simulink model "Simulation_der_Regler"  (R2016a)
settings: Solver=FixedStepAuto  StartTime=0  StopTime=10.0  FixedStep=T_s  RelTol=1e-3
values from neighbouring files (symbols this model uses):
  AD1 = expm(AC1*T_s)    [Regerlung_einer_WEA.m]
  AD2 = expm(AC2*T_s)    [Regerlung_einer_WEA.m]
  AD4 = expm(AC4*T_s)    [Regerlung_einer_WEA.m]
  BD1 = inv(AC1)*(expm(AC1*T_s)-I1)*BC1    [Regerlung_einer_WEA.m]
  BD2 = inv(AC2)*(expm(AC2*T_s)-I2)*BC2    [Regerlung_einer_WEA.m]
  BD2u = BD2(:,1:2)    [Regerlung_einer_WEA.m]
  BD4 = inv(AC4)*(expm(AC4*T_s)-I4)*BC4    [Regerlung_einer_WEA.m]
  C1 = zeors(s1*Nu,s1)    [OptimierungMitConstrains.m]    (also in Regerlung_einer_WEA.m = 1)
  C2 = zeors(s1*Nu,s1*Nu)    [OptimierungMitConstrains.m]    (also in Regerlung_einer_WEA.m = [1,0,0,0])
  C2full = eye(4)    [Regerlung_einer_WEA.m]
  C4 = [1,0,0,0,0,0,0,0 ... (first row only)    [Regerlung_einer_WEA.m]
  C4_base = [1,0,0,0,0,0,0,0 ... (first row only)    [Regerlung_einer_WEA.m]
  D1 = zeros(1,3)    [Regerlung_einer_WEA.m]
  D2 = zeros(1,3)    [Regerlung_einer_WEA.m]
  D2full = zeros(4,3)    [Regerlung_einer_WEA.m]
  D4 = zeros(5,3)    [Regerlung_einer_WEA.m]
  D4_base = zeros(6,3)    [Regerlung_einer_WEA.m]
  DeltaU2max = [8+pi/180+T_s,Inf]    [Regerlung_einer_WEA.m]
  DeltaU2min = [-8*pi/180*T_s,-Inf]    [Regerlung_einer_WEA.m]
  para_cntrl = struct()    [create_para_cntrl_5MWBaseline.m]    (also in para_cntrl_5MWBaseline.mat = )
  para_mdl = struct()    [Regerlung_einer_WEA.m]
  Qw2 = eye(100)*0.1    [Regerlung_einer_WEA.m]
  r2 = zeros(1,100)    [Regerlung_einer_WEA.m]
  ref_4 = [w_r_c;0;y_t_c;0;y_b_c]    [Regerlung_einer_WEA.m]
  Rw2 = eye(100)    [Regerlung_einer_WEA.m]
  T_g_c = 43093.5    [Regerlung_einer_WEA.m]
  T_s = 0.05    [Regerlung_einer_WEA.m]
  theta_c = 4*pi/180    (= 0.0698131700798)    [Regerlung_einer_WEA.m]
  U2max = [90*pi/180,43091.5]    [Regerlung_einer_WEA.m]
  U2min = [0,0]    [Regerlung_einer_WEA.m]
  v_c = 14.0    (= 14)    [Regerlung_einer_WEA.m]    (also in testinterpolation.m = [9,9.5,10,11,14,15,18,25])
  w_g_c = w_r_c*n_g    (= 122.9087)    [Regerlung_einer_WEA.m]
  w_r_c = 1.2671    [Regerlung_einer_WEA.m]
  Y2max = Inf    (= inf)    [Regerlung_einer_WEA.m]
  Y2min = 0    [Regerlung_einer_WEA.m]
  y_b_c = Datalogging.yb(s1(1))    [Regerlung_einer_WEA.m]
  y_t_c = Datalogging.yt(s1(1))    [Regerlung_einer_WEA.m]
undefined symbols (not defined in the file or in its folder): BD2ua, F2, F2a, G2, G2a, H2, H2a, v_t_c
libraries: mpclib x6
settings Model: Creator=pasca  LastModifiedBy=pasca
settings GRTTargetCC: GeneratePreprocessorConditionals=Use local settings

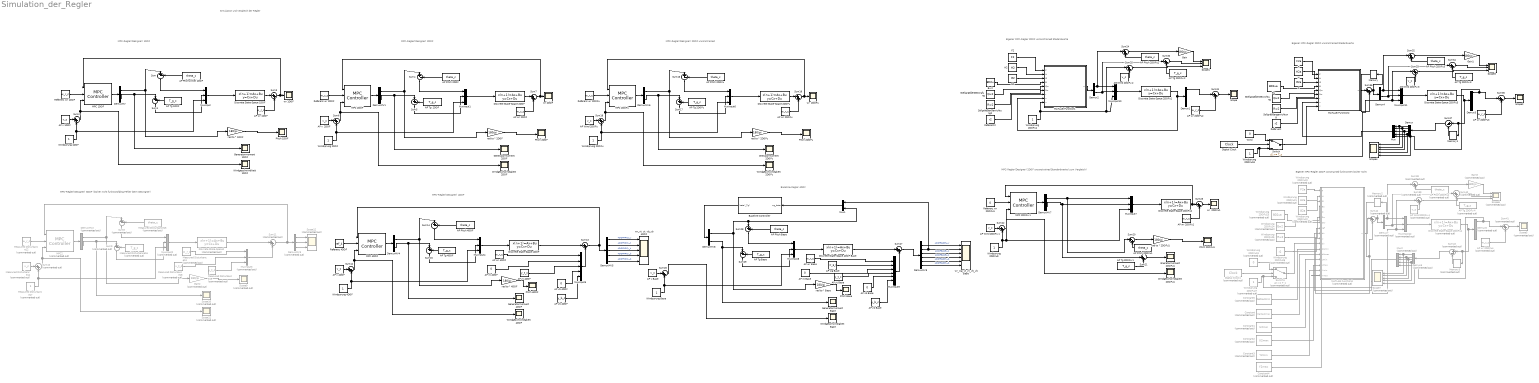
== system Simulation_der_Regler ==
  note: Eigener MPC-Regler 2DOF unconstrained Stadardwerte
  note: Simulation und Vergleich der Regler
  note: Baseline-Regler 4DOF
  note: MPC-Regler(Designer) 1DOF
  note: MPC-Regler(Designer) 2DOF
  note: MPC-Regler(Designer) 3DOF (bisher nicht funktionsfähig Fehler beim Desingner)
  note: MPC-Regler(Designer) 4DOF
  note: MPC-Regler(Designer) 2DOF unconstrained
  note: MPC-Regler(Designer) 2DOF unconstrained Standardwerte (zum Vergleich)
  note: Eigener MPC-Regler 2DOF unconstrained Stadardwerte
  note: Eigener MPC-Regler 2DOF constrained funktioniert bisher nicht
  " AP Ptichwinkel 1DOF " : Constant  Value=theta_c
  "AP Pitch 2DOF " : Constant  Value=theta_c
  AP Pitch 2DOFu{,1..3} (4 alike) : Constant  Value=theta_c
  AP Pitch 2DOFu4 : Constant  Commented=on  Value=theta_c
  AP Pitch 4DOF : Constant  Value=theta_c
  AP Pitch Base : Constant  Value=theta_c
  AP Tg  2DOF : Constant  Value=T_g_c
  "AP Tg 1DOF " : Constant  Value=T_g_c
  AP Tg 2DOFu {,1..3} (4 alike) : Constant  Value=T_g_c
  AP Tg 2DOFu 4 : Constant  Commented=on  Value=T_g_c
  AP Tg 4DOF : Constant  Value=T_g_c
  AP Tg Base : Constant  Value=T_g_c
  AP Wind 2DOFu {,1..3} (4 alike) : Constant  Value=v_c
  AP Wind 2DOFu 4 : Constant  Commented=on  Value=v_c
  AP v  2DOF : Constant  Value=v_c
  AP v 1DOF : Constant  Value=v_c
  "AP v 4DOF " : Constant  Value=v_c
  AP v Base : Constant  Value=v_c
  AP vb 4DOF : Constant  Value=0
  AP vb Base : Constant  Value=0
  AP vt 4DOF : Constant  Value=0
  AP vt Base : Constant  Value=0
  AP wg Base : Constant  Value=w_g_c
  "AP wr 1DOF " : Constant  Value=w_r_c
  "AP wr 2DOF " : Constant  Value=w_r_c
  AP wr 2DOFu{,1..3} (4 alike) : Constant  Value=w_r_c
  AP wr 2DOFu4 : Constant  Commented=on  Value=w_r_c
  AP wr 4DOF : Constant  Value=w_r_c
  AP wr Base : Constant  Value=w_r_c
  AP yb 4DOF : Constant  Value=y_b_c
  AP yb Base : Constant  Value=y_b_c
  AP yt 4DOF : Constant  Value=y_t_c
  AP yt Base : Constant  Value=y_t_c
  Baseline Controller : Subsystem
  "Bu " : Constant  Value=BD2ua
  Bu 2 : Constant  Value=BD2u
  Constant : Constant  Commented=on  Value=DeltaU2max
  Constant1 : Constant  Commented=on  Value=U2min
  Constant2 : Constant  Commented=on  Value=U2max
  Constant3 : Constant  Commented=on  Value=Y2min
  Constant4 : Constant  Commented=on  Value=Y2max
  Constant5 : Constant  Commented=on  Value=DeltaU2min
  Demux : Demux
  Demux1 : Demux
  Demux2 : Demux  Outputs=2
  Demux3 : Demux
  Demux4 : Demux  Outputs=2
  Demux5 : Demux  Commented=on
  Demux6 : Demux  Commented=on
  Demux7 : Demux  Commented=on  Outputs=2
  DemuxMV{,1,4,6..8} (6 alike) : Demux  Outputs=2
  DemuxMV2 : Demux  Commented=on  Outputs=2
  DemuxMV3 : Demux  Commented=on  Outputs=3
  DemuxMV5 : Demux  Outputs=5
  DemuxMV9 : Demux  Outputs=6
  Digital Clock : DigitalClock  SampleTime=T_s
  Digital Clock1 : DigitalClock  Commented=on  SampleTime=T_s
  "Discrete State-Space 1DOF " : DiscreteStateSpace  A=AD1  B=BD1  C=C1  D=D1  SampleTime=T_s
  Discrete State-Space 2DOF : DiscreteStateSpace  A=AD2  B=BD2  C=C2  D=D2  SampleTime=T_s
  Discrete State-Space 2DOFu : DiscreteStateSpace  A=AD2  B=BD2  C=C2  D=D2  SampleTime=T_s
  Discrete State-Space 2DOFu1 : DiscreteStateSpace  A=AD2  B=BD2  C=C2full  D=D2full  SampleTime=T_s
  Discrete State-Space 2DOFu2 : DiscreteStateSpace  A=AD2  B=BD2  C=C2  D=D2  SampleTime=T_s
  Discrete State-Space 2DOFu3 : DiscreteStateSpace  A=AD2  B=BD2  C=C2full  D=D2full  SampleTime=T_s
  Discrete State-Space 2DOFu4 : DiscreteStateSpace  Commented=on  A=AD2  B=BD2  C=C2full  D=D2full  SampleTime=T_s
  Discrete State-Space 4DOF : DiscreteStateSpace  A=AD4  B=BD4  C=C4  D=D4  SampleTime=T_s
  Discrete State-Space 4DOF Base : DiscreteStateSpace  A=AD4  B=BD4  C=C4_base  D=D4_base  SampleTime=T_s
  Discrete State-Space2 : DiscreteStateSpace  Commented=on  A=AD2  B=BD2  C=C2  D=D2  SampleTime=T_s
  "F " : Constant  Value=F2a
  F2 : Constant  Value=F2
  "G " : Constant  Value=G2a
  "G2 " : Constant  Value=G2
  Gain : Gain  Gain=180/pi
  Gain1 : Gain  Gain=180/pi
  Gain2 : Gain  Commented=on  Gain=180/pi
  Gain3 : Gain  Commented=on  Gain=180/pi
  "Generatormoment 1DOF " : Scope
  "Generatormoment 2DOF " : Scope
  Generatormoment 4DOF : Scope
  Generatormoment Base : Scope
  Gneratormoment 2DOFu : Scope
  Gneratormoment 2DOFu1 : Scope
  "H " : Constant  Value=H2a
  "H2 " : Constant  Value=H2
  MATLAB Function1 : MATLAB Function  TreatAsAtomicUnit=on
  MATLAB Function2 : MATLAB Function  TreatAsAtomicUnit=on
  MATLAB Function3 : MATLAB Function  Commented=on  TreatAsAtomicUnit=on
  "MPC 1DOF " : mpclib/MPC Controller  SCDEnableBlockLinearizationSpecification=on  mpcobj=mpc_F1  is_multiple=0  enable_value=0  return_u0=off  ref_from_ws=off  ref_signal_name=[]  ref_preview=off  md_from_ws=off  md_signal_name=[]  md_preview=off  from_project=off  project_file=MPCtask.mat  md_inport=on  mv_inport=off  cost_outport=off  return_sequence=off  return_qpstatus=off  return_state=off  state_inport=off  lims_inport=off  ywt_inport=off  is_designfromscratch=0  uwt_inport=off  duwt_inport=off  rhoeps_inport=off  uref_inport=off  n_ts=0.05  n_mv=2  n_md=1  n_ud=0  n_mo=1  n_uo=0  BlockDataType=double  SampleTimeInherited=off  switch_inport=off
  "MPC 2DOF " : mpclib/MPC Controller  SCDEnableBlockLinearizationSpecification=on  mpcobj=mpc_F2  is_multiple=0  enable_value=0  return_u0=off  ref_from_ws=off  ref_signal_name=[]  ref_preview=off  md_from_ws=off  md_signal_name=[]  md_preview=off  from_project=off  project_file=MPCtask.mat  md_inport=on  mv_inport=off  cost_outport=off  return_sequence=off  return_qpstatus=off  return_state=off  state_inport=off  lims_inport=off  ywt_inport=off  is_designfromscratch=0  uwt_inport=off  duwt_inport=off  rhoeps_inport=off  uref_inport=off  n_ts=0.05  n_mv=2  n_md=1  n_ud=0  n_mo=1  n_uo=0  BlockDataType=double  SampleTimeInherited=off  switch_inport=off
  "MPC 2DOFu " : mpclib/MPC Controller  SCDEnableBlockLinearizationSpecification=on  mpcobj=mpc_F2_u  is_multiple=0  enable_value=0  return_u0=off  ref_from_ws=off  ref_signal_name=[]  ref_preview=off  md_from_ws=off  md_signal_name=[]  md_preview=off  from_project=off  project_file=MPCtask.mat  md_inport=on  mv_inport=off  cost_outport=off  return_sequence=off  return_qpstatus=off  return_state=off  state_inport=off  lims_inport=off  ywt_inport=off  is_designfromscratch=0  uwt_inport=off  duwt_inport=off  rhoeps_inport=off  uref_inport=off  n_ts=0.05  n_mv=2  n_md=1  n_ud=0  n_mo=1  n_uo=0  BlockDataType=double  SampleTimeInherited=off  switch_inport=off
  MPC 2DOFu 1 : mpclib/MPC Controller  SCDEnableBlockLinearizationSpecification=on  mpcobj=mpc_F2_us  is_multiple=0  enable_value=0  return_u0=off  ref_from_ws=off  ref_signal_name=[]  ref_preview=off  md_from_ws=off  md_signal_name=[]  md_preview=off  from_project=off  project_file=MPCtask.mat  md_inport=on  mv_inport=off  cost_outport=off  return_sequence=off  return_qpstatus=off  return_state=off  state_inport=off  lims_inport=off  ywt_inport=off  is_designfromscratch=0  uwt_inport=off  duwt_inport=off  rhoeps_inport=off  uref_inport=off  n_ts=0.05  n_mv=2  n_md=1  n_ud=0  n_mo=1  n_uo=0  BlockDataType=double  SampleTimeInherited=off  switch_inport=off
  MPC 4DOF : mpclib/MPC Controller  SCDEnableBlockLinearizationSpecification=on  mpcobj=mpc_F4  is_multiple=0  enable_value=0  return_u0=off  ref_from_ws=off  ref_signal_name=[]  ref_preview=off  md_from_ws=off  md_signal_name=[]  md_preview=off  from_project=off  project_file=MPCtask.mat  md_inport=on  mv_inport=off  cost_outport=off  return_sequence=off  return_qpstatus=off  return_state=off  state_inport=off  lims_inport=off  ywt_inport=off  is_designfromscratch=0  uwt_inport=off  duwt_inport=off  rhoeps_inport=off  uref_inport=off  n_ts=0.05  n_mv=2  n_md=1  n_ud=0  n_mo=5  n_uo=0  BlockDataType=double  SampleTimeInherited=off  switch_inport=off
  MPC2 : mpclib/MPC Controller  Commented=on  SCDEnableBlockLinearizationSpecification=on  mpcobj=mpc_F1  is_multiple=0  enable_value=0  return_u0=off  ref_from_ws=off  ref_signal_name=[]  ref_preview=off  md_from_ws=off  md_signal_name=[]  md_preview=off  from_project=off  project_file=MPCtask.mat  md_inport=on  mv_inport=off  cost_outport=off  return_sequence=off  return_qpstatus=off  return_state=off  state_inport=off  lims_inport=off  ywt_inport=off  is_designfromscratch=0  uwt_inport=off  duwt_inport=off  rhoeps_inport=off  uref_inport=off  n_ts=0.05  n_mv=2  n_md=1  n_ud=0  n_mo=1  n_uo=0  BlockDataType=double  SampleTimeInherited=off  switch_inport=off
  Measured Disturbance12 : Constant  Commented=on  Value=w_r_c
  Measured Disturbance13 : Constant  Commented=on  Value=w_r_c
  Measured Disturbance14 : Constant  Commented=on  Value=v_c
  Measured Disturbance15 : Constant  Commented=on  Value=theta_c
  Measured Disturbance16 : Constant  Commented=on  Value=T_g_c
  Measured Disturbance17 : Constant  Commented=on
  Measured Disturbance18 : Constant  Commented=on  Value=v_t_c
  Measured Disturbance19 : Constant  Commented=on  Value=y_t_c
  Memory : Memory
  Memory1 : Memory
  Memory2 : Memory  Commented=on
  Memory3 : Memory  Commented=on
  Mux : Mux  Inputs=5
  Mux1 : Mux  Inputs=2
  Mux2 : Mux  Commented=on  Inputs=5
  MuxInput{,1,4,6..8,10..11} (8 alike) : Mux  Inputs=3
  MuxInput12 : Mux  Commented=on  Inputs=3
  MuxInput2 : Mux  Commented=on  Inputs=3
  MuxInput3 : Mux  Commented=on  Inputs=3
  MuxInput5 : Mux  Inputs=5
  MuxInput9 : Mux  Inputs=6
  "Pitch 1DOF " : Scope
  Pitch 2DOFu : Scope
  Pitch 2DOFu1 : Scope
  Pitch 4DOF : Scope
  Pitch Base : Scope
  "Ptich 2DOF " : Scope
  Refer enz : Constant  Value=r2
  Referenz 4DOF : Constant  Value=ref_4
  "Referenz wr 1DOF " : Constant  Value=w_r_c
  "Referenz wr 2DOF " : Constant  Value=w_r_c
  Referenz wr 2DOFu : Constant  Value=w_r_c
  Referenz wr 2DOFu1 : Constant  Value=0
  "Referenz2 " : Constant  Value=r2
  Scope : Scope
  Scope1 : Scope  NumInputPorts=3
  Scope{5,9..11} (4 alike) : Scope  Commented=on
  Scope12 : Scope  Commented=on  NumInputPorts=3
  Scope2 : Scope
  Scope3 : Scope  NumInputPorts=3
  Scope4 : Scope  NumInputPorts=5
  Scope6 : Scope  Commented=on  NumInputPorts=3
  Scope7 : Scope  Commented=on  NumInputPorts=5
  SollgräößenGewichtung2 : Constant  Value=Rw2
  Sollgräößengewichtung : Constant  Value=Rw2
  StellgräößenBestrafung : Constant  Value=Qw2
  "StellgräößenGewichtung " : Constant  Value=Qw2
  Sum{,1,4..5,14..17,28..29,37} (11 alike) : Sum  Inputs=|+-
  Sum{10..11,38..42} (7 alike) : Sum  Commented=on  Inputs=|++
  Sum{2..3,6..7,12..13,18..27,30..36} (23 alike) : Sum  Inputs=|++
  Sum43 : Sum  Commented=on  Inputs=|+-
  Sum8 : Sum  Commented=on  Inputs=|+-
  Sum9 : Sum  Commented=on  Inputs=|+-
  Switch : Switch  Threshold=T_s
  Switch1 : Switch  Commented=on  Threshold=T_s
  "Wind " : Constant  Value=0  VectorParams1D=off  SampleTime=T_s
  "Windgeschwindigkeit 2DOF " : Scope
  Windgeschwindigkeit 2DOFu : Scope
  Windgeschwindigkeit 2DOFu1 : Scope
  Windgeschwindigkeit 4DOF : Scope
  Windgeschwindigkeit Base : Scope
  "Windgeschwindikeit 1DOF " : Scope
  "Windsprung 1DOF " : Constant
  "Windsprung 2DOF " : Constant
  Windsprung 2DOFu : Constant
  Windsprung 2DOFu1 : Constant
  Windsprung 2DOFu18 : Constant  VectorParams1D=off  SampleTime=T_s
  Windsprung 2DOFu19 : Constant  Commented=on  Value=0  VectorParams1D=off  SampleTime=T_s
  Windsprung 2DOFu20 : Constant  Commented=on  Value=F2a
  Windsprung 2DOFu21 : Constant  Commented=on  Value=H2a
  Windsprung 2DOFu22 : Constant  Commented=on  Value=G2a
  Windsprung 2DOFu23 : Constant  Commented=on  Value=BD2ua
  Windsprung 2DOFu24 : Constant  Commented=on  Value=Qw2
  Windsprung 2DOFu25 : Constant  Commented=on  Value=Rw2
  Windsprung 2DOFu26 : Constant  Commented=on  Value=r2
  Windsprung 2DOFu27 : Constant  Commented=on  VectorParams1D=off  SampleTime=T_s
  Windsprung 2DOFu9 : Constant
  Windsprung 4DOF : Constant
  Windsprung Base : Constant
  "rad to ° 1DOF " : Gain  Gain=180/pi
  "rad to ° 2DOF " : Gain  Gain=180/pi
  rad to ° 2DOFu : Gain  Gain=180/pi
  rad to ° 2DOFu1 : Gain  Gain=180/pi
  rad to ° 4DOF : Gain  Gain=180/pi
  rad to ° Base : Gain  Gain=180/pi
  wr  2DOFu : Scope
  wr  2DOFu1 : Scope
  "wr 1DOF " : Scope
  wr 2DOF : Scope
  wr_vt_yt_vb_yb 4DOF : Scope  NumInputPorts=5
  wr_wg_vt_yt_vb_yb Base : Scope  NumInputPorts=6
  wires:
  "Referenz wr 1DOF "/1 -> "MPC 1DOF "/2
  "MPC 1DOF "/1 -> DemuxMV/1
  MuxInput/1 -> "Discrete State-Space 1DOF "/1
  Sum/1 -> MuxInput/1
  DemuxMV/1 -> Sum/1, "rad to ° 1DOF "/1
  " AP Ptichwinkel 1DOF "/1 -> Sum/2
  DemuxMV/2 -> "Generatormoment 1DOF "/1, Sum1/1
  Sum1/1 -> MuxInput/2
  "AP Tg 1DOF "/1 -> Sum1/2
  AP v 1DOF/1 -> Sum2/1
  Sum2/1 -> "Windgeschwindikeit 1DOF "/1, "MPC 1DOF "/3
  "Windsprung 1DOF "/1 -> MuxInput/3, Sum2/2
  "Discrete State-Space 1DOF "/1 -> Sum3/1
  "AP wr 1DOF "/1 -> Sum3/2
  Sum3/1 -> "wr 1DOF "/1, "MPC 1DOF "/1
  "rad to ° 1DOF "/1 -> "Pitch 1DOF "/1
  "Referenz wr 2DOF "/1 -> "MPC 2DOF "/2
  "MPC 2DOF "/1 -> DemuxMV1/1
  MuxInput1/1 -> Discrete State-Space 2DOF/1
  Sum4/1 -> MuxInput1/1
  DemuxMV1/1 -> Sum4/1, "rad to ° 2DOF "/1
  "AP Pitch 2DOF "/1 -> Sum4/2
  DemuxMV1/2 -> "Generatormoment 2DOF "/1, Sum5/1
  Sum5/1 -> MuxInput1/2
  AP Tg  2DOF/1 -> Sum5/2
  AP v  2DOF/1 -> Sum6/1
  Sum6/1 -> "Windgeschwindigkeit 2DOF "/1, "MPC 2DOF "/3
  "Windsprung 2DOF "/1 -> MuxInput1/3, Sum6/2
  Discrete State-Space 2DOF/1 -> Sum7/1
  "AP wr 2DOF "/1 -> Sum7/2
  Sum7/1 -> wr 2DOF/1, "MPC 2DOF "/1
  "rad to ° 2DOF "/1 -> "Ptich 2DOF "/1
  Measured Disturbance12/1 -> MPC2/2
  MPC2/1 -> DemuxMV2/1
  MuxInput2/1 -> Discrete State-Space2/1
  Sum8/1 -> MuxInput2/1
  DemuxMV2/1 -> Sum8/1, Gain2/1
  Measured Disturbance15/1 -> Sum8/2
  DemuxMV2/2 -> Scope10/1, Sum9/1
  Sum9/1 -> MuxInput2/2
  Measured Disturbance16/1 -> Sum9/2
  Measured Disturbance14/1 -> Sum10/1
  Sum10/1 -> Scope11/1, MPC2/3
  Measured Disturbance17/1 -> MuxInput2/3, Sum10/2
  Sum11/1 -> DemuxMV3/1, MPC2/1
  Gain2/1 -> Scope9/1
  Discrete State-Space2/1 -> Sum11/1
  MuxInput3/1 -> Sum11/2
  DemuxMV3/1 -> Scope12/1
  DemuxMV3/2 -> Scope12/2
  DemuxMV3/3 -> Scope12/3
  Measured Disturbance13/1 -> MuxInput3/1
  Measured Disturbance19/1 -> MuxInput3/3
  Measured Disturbance18/1 -> MuxInput3/2
  Referenz 4DOF/1 -> MPC 4DOF/2
  MPC 4DOF/1 -> DemuxMV4/1
  MuxInput4/1 -> Discrete State-Space 4DOF/1
  Sum14/1 -> MuxInput4/1
  DemuxMV4/1 -> Sum14/1, rad to ° 4DOF/1
  AP Pitch 4DOF/1 -> Sum14/2
  DemuxMV4/2 -> Generatormoment 4DOF/1, Sum15/1
  Sum15/1 -> MuxInput4/2
  AP Tg 4DOF/1 -> Sum15/2
  "AP v 4DOF "/1 -> Sum12/1
  Sum12/1 -> Windgeschwindigkeit 4DOF/1, MPC 4DOF/3
  Windsprung 4DOF/1 -> MuxInput4/3, Sum12/2
  Sum13/1 -> DemuxMV5/1, MPC 4DOF/1
  rad to ° 4DOF/1 -> Pitch 4DOF/1
  Discrete State-Space 4DOF/1 -> Sum13/1
  MuxInput5/1 -> Sum13/2
  DemuxMV5/2 -> wr_vt_yt_vb_yb 4DOF/2  "4DOFMPCv_t"
  DemuxMV5/3 -> wr_vt_yt_vb_yb 4DOF/3  "4DOFMPCy_t"
  AP wr 4DOF/1 -> MuxInput5/1
  AP yt 4DOF/1 -> MuxInput5/3
  AP vt 4DOF/1 -> MuxInput5/2
  DemuxMV5/4 -> wr_vt_yt_vb_yb 4DOF/4  "4DOFMPCv_b"
  DemuxMV5/5 -> wr_vt_yt_vb_yb 4DOF/5  "4DOFMPCy_b"
  AP vb 4DOF/1 -> MuxInput5/4
  AP yb 4DOF/1 -> MuxInput5/5
  Referenz wr 2DOFu/1 -> "MPC 2DOFu "/2
  "MPC 2DOFu "/1 -> DemuxMV6/1
  MuxInput6/1 -> Discrete State-Space 2DOFu/1
  Sum16/1 -> MuxInput6/1
  DemuxMV6/1 -> Sum16/1, rad to ° 2DOFu/1
  AP Pitch 2DOFu/1 -> Sum16/2
  DemuxMV6/2 -> Gneratormoment 2DOFu/1, Sum17/1
  Sum17/1 -> MuxInput6/2
  "AP Tg 2DOFu "/1 -> Sum17/2
  "AP Wind 2DOFu "/1 -> Sum18/1
  Sum18/1 -> Windgeschwindigkeit 2DOFu/1, "MPC 2DOFu "/3
  Windsprung 2DOFu/1 -> MuxInput6/3, Sum18/2
  Discrete State-Space 2DOFu/1 -> Sum19/1
  AP wr 2DOFu/1 -> Sum19/2
  Sum19/1 -> wr  2DOFu/1, "MPC 2DOFu "/1
  rad to ° 2DOFu/1 -> Pitch 2DOFu/1
  MuxInput8/1 -> Discrete State-Space 4DOF Base/1
  Sum28/1 -> MuxInput8/1
  DemuxMV8/1 -> rad to ° Base/1, Sum28/1, Mux1/2
  AP Pitch Base/1 -> Sum28/2
  DemuxMV8/2 -> Generatormoment Base/1, Sum29/1
  Sum29/1 -> MuxInput8/2
  AP Tg Base/1 -> Sum29/2
  AP v Base/1 -> Sum26/1
  Sum26/1 -> Windgeschwindigkeit Base/1
  Windsprung Base/1 -> MuxInput8/3, Sum26/2
  Sum27/1 -> DemuxMV9/1
  rad to ° Base/1 -> Pitch Base/1
  Discrete State-Space 4DOF Base/1 -> Sum27/1
  MuxInput9/1 -> Sum27/2
  DemuxMV9/1 -> wr_wg_vt_yt_vb_yb Base/1  "4DOFBASEw_r"
  DemuxMV9/2 -> Mux1/1, wr_wg_vt_yt_vb_yb Base/2
  DemuxMV9/3 -> wr_wg_vt_yt_vb_yb Base/3  "4DOFBASEv_t"
  AP wr Base/1 -> MuxInput9/1
  DemuxMV9/4 -> wr_wg_vt_yt_vb_yb Base/4  "4DOFBASEy_t"
  DemuxMV9/5 -> wr_wg_vt_yt_vb_yb Base/5  "4DOFBASEv_b"
  Baseline Controller/1(beta*_Tg*) -> DemuxMV8/1
  DemuxMV9/6 -> wr_wg_vt_yt_vb_yb Base/6  "4DOFBASEy_b"
  AP vt Base/1 -> MuxInput9/3
  AP yt Base/1 -> MuxInput9/4
  AP vb Base/1 -> MuxInput9/5
  AP yb Base/1 -> MuxInput9/6
  AP wg Base/1 -> MuxInput9/2
  Mux1/1 -> Baseline Controller/1(wg_beta)
  MuxInput10/1 -> Discrete State-Space 2DOFu1/1
  MATLAB Function1/1(u) -> Demux2/1
  Demux2/2 -> Sum30/1, MuxInput10/2
  Windsprung 2DOFu1/1 -> Sum25/1, MuxInput10/3, MATLAB Function1/9(v)
  Discrete State-Space 2DOFu1/1 -> MATLAB Function1/8(x), Demux1/1
  F2/1 -> MATLAB Function1/1(F)
  "H2 "/1 -> MATLAB Function1/2(H)
  "G2 "/1 -> MATLAB Function1/3(G)
  Bu 2/1 -> MATLAB Function1/4(B)
  StellgräößenBestrafung/1 -> MATLAB Function1/5(Qw)
  SollgräößenGewichtung2/1 -> MATLAB Function1/6(Rw)
  "Referenz2 "/1 -> MATLAB Function1/7(r)
  Demux2/1 -> Sum24/1, MuxInput10/1
  Gain/1 -> Scope1/1
  Referenz wr 2DOFu1/1 -> MPC 2DOFu 1/2
  MPC 2DOFu 1/1 -> DemuxMV7/1
  MuxInput7/1 -> Discrete State-Space 2DOFu2/1
  DemuxMV7/1 -> Sum20/1, MuxInput7/1
  DemuxMV7/2 -> Sum21/1, MuxInput7/2
  AP Wind 2DOFu 1/1 -> Sum22/1
  Sum22/1 -> Windgeschwindigkeit 2DOFu1/1
  Windsprung 2DOFu9/1 -> MuxInput7/3, MPC 2DOFu 1/3, Sum22/2
  Discrete State-Space 2DOFu2/1 -> MPC 2DOFu 1/1, Sum23/1
  AP wr 2DOFu1/1 -> Sum23/2
  Sum23/1 -> wr  2DOFu1/1
  rad to ° 2DOFu1/1 -> Pitch 2DOFu1/1
  Sum24/1 -> Gain/1
  AP Pitch 2DOFu2/1 -> Sum24/2
  AP Wind 2DOFu 2/1 -> Sum25/2
  Sum25/1 -> Scope1/3
  Sum30/1 -> Scope1/2
  AP Tg 2DOFu 2/1 -> Sum30/2
  Sum31/1 -> Scope/1
  AP wr 2DOFu2/1 -> Sum31/2
  Demux1/1 -> Sum31/1
  Sum20/1 -> rad to ° 2DOFu1/1
  Sum21/1 -> Gneratormoment 2DOFu1/1
  AP Pitch 2DOFu1/1 -> Sum20/2
  AP Tg 2DOFu 1/1 -> Sum21/2
  MuxInput11/1 -> Discrete State-Space 2DOFu3/1
  Demux4/2 -> Sum34/1, MuxInput11/2
  Discrete State-Space 2DOFu3/1 -> Memory1/1, Sum37/1, Demux3/1
  "F "/1 -> MATLAB Function2/1(F)
  "H "/1 -> MATLAB Function2/2(H)
  "G "/1 -> MATLAB Function2/3(G)
  "Bu "/1 -> MATLAB Function2/4(B)
  "StellgräößenGewichtung "/1 -> MATLAB Function2/5(Qw)
  Sollgräößengewichtung/1 -> MATLAB Function2/6(Rw)
  Refer enz/1 -> MATLAB Function2/7(r)
  Demux4/1 -> Sum32/1, MuxInput11/1
  Gain1/1 -> Scope3/1
  Sum32/1 -> Gain1/1
  AP Pitch 2DOFu3/1 -> Sum32/2
  AP Wind 2DOFu 3/1 -> Sum33/2
  Sum33/1 -> Scope3/3
  Sum34/1 -> Scope3/2
  AP Tg 2DOFu 3/1 -> Sum34/2
  Sum35/1 -> Scope2/1
  AP wr 2DOFu3/1 -> Sum35/2
  MATLAB Function2/1(u) -> Sum36/1
  Sum36/1 -> Memory/1, Demux4/1
  Memory/1 -> Sum36/2
  Sum37/1 -> Demux/1
  Demux/1 -> Scope4/1, Mux/1
  Demux/2 -> Scope4/2, Mux/2
  Demux/3 -> Scope4/3, Mux/3
  Demux/4 -> Scope4/4, Mux/4
  Mux/1 -> MATLAB Function2/8(x)
  Demux3/1 -> Scope4/5, Mux/5, Sum35/1
  Memory1/1 -> Sum37/2
  Switch/1 -> MATLAB Function2/9(v)
  "Wind "/1 -> Switch/1
  Windsprung 2DOFu18/1 -> Sum33/1, MuxInput11/3, Switch/3
  Digital Clock/1 -> Switch/2
  MuxInput12/1 -> Discrete State-Space 2DOFu4/1
  Demux7/2 -> Sum40/1, MuxInput12/2
  Discrete State-Space 2DOFu4/1 -> Memory3/1, Sum43/1, Demux6/1
  Windsprung 2DOFu20/1 -> MATLAB Function3/1(F)
  Windsprung 2DOFu21/1 -> MATLAB Function3/2(H)
  Windsprung 2DOFu22/1 -> MATLAB Function3/3(G)
  Windsprung 2DOFu23/1 -> MATLAB Function3/4(Bu)
  Windsprung 2DOFu24/1 -> MATLAB Function3/7(Qw)
  Windsprung 2DOFu25/1 -> MATLAB Function3/6(Rw)
  Windsprung 2DOFu26/1 -> MATLAB Function3/8(ref)
  Demux7/1 -> Sum38/1, MuxInput12/1
  Gain3/1 -> Scope6/1
  Sum38/1 -> Gain3/1
  AP Pitch 2DOFu4/1 -> Sum38/2
  AP Wind 2DOFu 4/1 -> Sum39/2
  Sum39/1 -> Scope6/3
  Sum40/1 -> Scope6/2
  AP Tg 2DOFu 4/1 -> Sum40/2
  Sum41/1 -> Scope5/1
  AP wr 2DOFu4/1 -> Sum41/2
  MATLAB Function3/1(u) -> Sum42/1
  Sum42/1 -> Memory2/1, Demux7/1
  Memory2/1 -> Sum42/2, MATLAB Function3/10("u ")
  Sum43/1 -> Demux5/1
  Demux5/1 -> Scope7/1, Mux2/1
  Demux5/2 -> Scope7/2, Mux2/2
  Demux5/3 -> Scope7/3, Mux2/3
  Demux5/4 -> Scope7/4, Mux2/4
  Mux2/1 -> MATLAB Function3/9(dx)
  Demux6/1 -> Scope7/5, Mux2/5, Sum41/1
  Memory3/1 -> Sum43/2
  Windsprung 2DOFu19/1 -> Switch1/1
  Windsprung 2DOFu27/1 -> Sum39/1, MuxInput12/3, Switch1/3
  Digital Clock1/1 -> Switch1/2
  Switch1/1 -> MATLAB Function3/11(dv)
  Constant5/1 -> MATLAB Function3/12(dUmin)
  Constant/1 -> MATLAB Function3/13(dUmax)
  Constant1/1 -> MATLAB Function3/14(Umin)
  Constant2/1 -> MATLAB Function3/15(Umax)
  Constant3/1 -> MATLAB Function3/16(Ymin)
  Constant4/1 -> MATLAB Function3/17(Ymax)
  DemuxMV5/1 -> wr_vt_yt_vb_yb 4DOF/1  "4DOFMPCw_r"

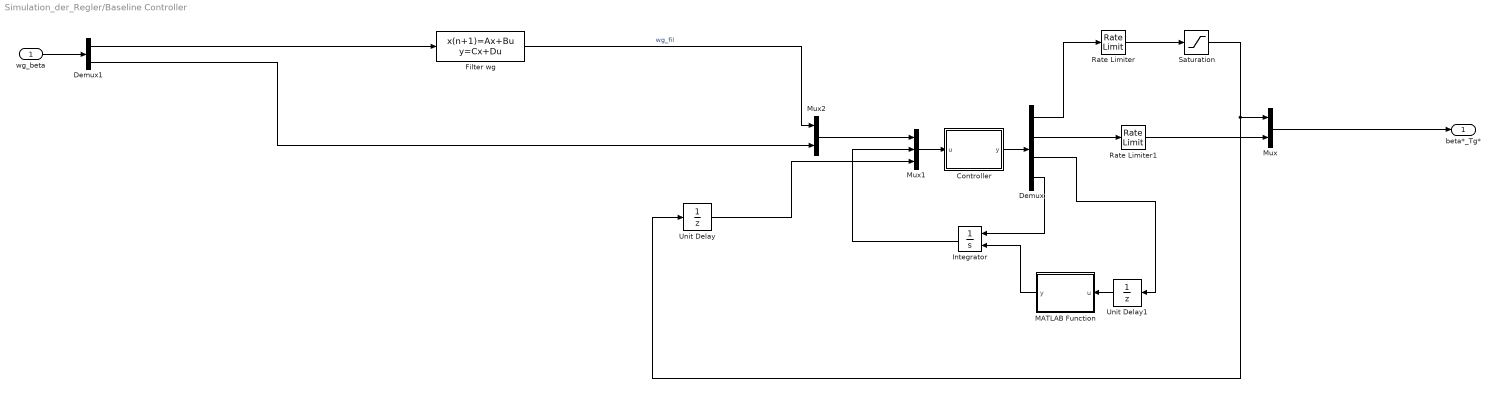
== system Simulation_der_Regler/Baseline Controller ==
  wg_beta : Inport
  Controller : MATLAB Function  TreatAsAtomicUnit=on
  Demux : Demux
  Demux1 : Demux  Outputs=2
  Filter wg : DiscreteStateSpace  A=exp(-2*pi*para_mdl.dT*para_cntrl.filter.fc)  B=1-exp(-2*pi*para_mdl.dT*para_cntrl.filter.fc)  C=exp(-2*pi*para_mdl.dT*para_cntrl.filter.fc)  D=1-exp(-2*pi*para_mdl.dT*para_cntrl.filter.fc)  X0=para_cntrl.ref.wg_d  SampleTime=para_mdl.dT
  Integrator : Integrator  ExternalReset=rising  InitialCondition=para_cntrl.initial.int_PCntrl
  MATLAB Function : MATLAB Function  TreatAsAtomicUnit=on
  Mux : Mux  Inputs=2
  Mux1 : Mux  Inputs=3
  Mux2 : Mux  Inputs=2
  Rate Limiter : RateLimiter  RisingSlewLimit=para_cntrl.limits.beta_rate/180*pi  FallingSlewLimit=-para_cntrl.limits.beta_rate/180*pi  SampleTimeMode=inherited
  Rate Limiter1 : RateLimiter  RisingSlewLimit=para_cntrl.limits.Tg_rate  FallingSlewLimit=-para_cntrl.limits.Tg_rate  SampleTimeMode=inherited
  Saturation : Saturate  UpperLimit=90/180*pi  LowerLimit=0
  Unit Delay : UnitDelay  SampleTime=para_mdl.dT
  Unit Delay1 : UnitDelay  SampleTime=para_mdl.dT
  beta*_Tg* : Outport
  wires:
  Rate Limiter1/1 -> Mux/2
  Demux/1 -> Rate Limiter/1
  Mux1/1 -> Controller/1(u)
  Demux/4 -> Integrator/1
  Mux/1 -> beta*_Tg*/1
  Demux/2 -> Rate Limiter1/1
  Controller/1(y) -> Demux/1
  Demux/3 -> Unit Delay1/1
  Integrator/1 -> Mux1/2
  wg_beta/1 -> Demux1/1
  Unit Delay/1 -> Mux1/3
  Demux1/2 -> Mux2/2
  Mux2/1 -> Mux1/1
  Filter wg/1 -> Mux2/1  "wg_fil"
  MATLAB Function/1(y) -> Integrator/2
  Unit Delay1/1 -> MATLAB Function/1(u)
  Rate Limiter/1 -> Saturation/1
  Saturation/1 -> Unit Delay/1, Mux/1
  Demux1/1 -> Filter wg/1

== matlab function Simulation_der_Regler/Baseline Controller/Controller ==
  data: u input size=4,1; y output; para_cntrl parameter
function y = fcn(u,para_cntrl)
% Regler für den gesamten Arbeitsbereich der Windturbine, für eine
% Beschreibung der Reglerparameter und verwendeten Arbeitspunkte: create_para_cntrl_5MWBaseline.m

% --------------------------------------------------- read inputs
% the input size of u is determined in the simulink model explorer (otherwise Simulink produces errors)

wg = u(1); % in [rad/s]; filtered
beta = u(2)/180*pi; % in [deg]/180*pi = [rad] not used, actually the pitch angle one step before is used for gain scheduling and decision on control region

int_delta_wg = u(3); % integral of the error; used for the pitch controller
beta_prev = u(4);% [rad], previous value of beta_d

% --------------------------------------------------- 

delta_wg = 0;   % set delta_wg to 0 to stop integrating if not in region (3) --> in region 3 delta_wg is defined again

wg_d    = para_cntrl.ref.wg_d;                                 % Solldrehzahl Generator in rad/s
Tgmax   = para_cntrl.ref.Tgmax;                                % max. Generator torque

Kopt =  para_cntrl.Kopt;                                              % Region 2 optimal Torque Open Loop Tg = Kopt*wr^2; kopt from NREL FAST Description
Tg_slope15 = para_cntrl.Tg_slope15;                                   % Region 15, linear ramp from w_cut_in to region 2
Tg_slope25 = para_cntrl.Tg_slope25;%Tgmax/(wg_d-.9*wg_d);
Tgx = para_cntrl.Tgx;

wg_SP_15                  = para_cntrl.ref.wg_SP_15;                    % wg Setpoint for Region 1.5
wg_SP_2                   = para_cntrl.ref.wg_SP_2;                     % wg Setpoint for Region 2
wg_SP_25                  = para_cntrl.ref.wg_SP_25;                    % wg Setpoint for Region 2.5
wg_SP_3                   = para_cntrl.ref.wg_SP_3;                     % wg Setpoint for Region 2.5

% Figure out which Region we are in:                                                                             
if wg < wg_SP_15 && (beta_prev < 1/180*pi) % Region 1
    reg = 1;
elseif wg < wg_SP_2 && (beta_prev < 1/180*pi) % Region 1,5
    reg = 2;
elseif wg < wg_SP_25 && (beta_prev < 1/180*pi) % Region 2
    reg = 3;
elseif (wg < wg_SP_3) && (beta_prev < 1/180*pi)% Region 2,5; NREL 5MW WT Description: 99% of the nominal speed; conditional statement on (beta_prev < 1/180*pi) also from FAST
    reg = 4;
else 
    reg = 5; % Region 3
end

% --------------- set the control output - overwritten in the switch case statement, needed for simulink
uc = [0 ; Tgmax]; 
% ---------------

switch reg 
    case 1 % Region 1
        uc = [0 ; 0];
    case 2 % Region 1.5
        Tg = Tg_slope15 * (wg - wg_SP_15);
        uc = [0 ; Tg];
    case 3 % Region 2
        Tg = Kopt*(wg*30/pi)^2; % Kopt is in [Nm/rpm^2]
        uc = [0 ; Tg];
    case 4 % Region 2.5
        Tg = Tg_slope25*wg + Tgx; % Tg_slope25 in [Nm/rad/s]
        if Tg > Tgmax
            disp(Tg-Tgmax)
            Tg = Tgmax;
        end
        uc = [0 ; Tg];
    case 5 % Region 3
        
        % calculation of the Pitch Angle
        betak = para_cntrl.ref.betak;    % in combination with beta_previous determines the scheduling
        Kp = para_cntrl.Kp0*1/(1+beta_prev/betak);
        Ki = para_cntrl.Ki0*1/(1+beta_prev/betak);
        delta_wg = (wg-wg_d);
        betad = (Kp*delta_wg + Ki*int_delta_wg); % in [rad]
        
        %calculation of the torque
        if wg < wg_d 
            Tg = Tg_slope25*wg + Tgx;
            if Tg < (Tg_slope25*.99*wg_d + Tgx)
                Tg = Tg_slope25*.99*wg_d + Tgx;
            end
        elseif para_cntrl.var_Trq_Reg3 == 1 
            Tg = para_cntrl.para.P0/wg;
        else
            Tg = Tgmax;
        end
        uc = [betad ; Tg]; 
end
y = [uc ; reg ; delta_wg];

== matlab function Simulation_der_Regler/MATLAB Function2 ==
  data: F input; u output; H input; G input; B input; Qw input; Rw input; r input; x input; v input
function u = GetOptimaleStellgroese(F,H,G,B,Qw,Rw,r,x,v)
s1=size(B,2);
s2=size(G,2);
v_vec=ones(s2,1)*v;
u_work= inv((H'*Rw*H)+Qw)*H'*Rw*(r-(F*x+G*v_vec));
u=u_work(1:s1);
end

== matlab function Simulation_der_Regler/Baseline Controller/MATLAB Function ==
  data: u input; y output
function y = fcn(u)
%#codegen
if u < 5
    y = 1;
else 
    y = 0;
end

== matlab function Simulation_der_Regler/MATLAB Function1 ==
  data: F input; u output; H input; G input; B input; Qw input; Rw input; r input; x input; v input
function u = GetOptimaleStellgroese(F,H,G,B,Qw,Rw,r,x,v)
s1=size(B,2);
s2=size(G,2);
v_vec=ones(s2,1)*v;
u_work= inv((H'*Rw*H)+Qw)*H'*Rw*(r-(F*x+G*v_vec));
u=u_work(1:s1);
end

== matlab function Simulation_der_Regler/MATLAB Function3 ==
  data: F input; u output; H input; G input; Bu input; C input; Rw input; Qw input; ref input; dx input; u input; dv input; dUmin input; dUmax input; Umin input; Umax input; Ymin input; Ymax input
function u=OptimierungMitConstrains(F,H,G,Bu,C,Rw,Qw,ref,dx,u,dv,dUmin,dUmax,Umin,Umax,Ymin,Ymax)
coder.extrinsic('quadprog','optimoptions');
s1=size(Bu,2);
s2=size(G,2);
s3=size(C,1);
Nu=size(H,2)/s1;
N2=size(H,1)/s3;
v_vec=ones(s2,1)*dv;
E=2*(H'*Rw*H+Qw);
f=2*H'*Rw*(ref-F*dx-G*v_vec);
gamma1min=zeros(s1*Nu,1);
gamma1max=zeros(s1*Nu,1);
gamma2min=zeros(s1*Nu,1);
gamma2max=zeros(s1*Nu,1);
for k=0:s1:(Nu-1)*s1
  gamma1min(k+1:k+s1,1)=Umin;
  gamma1max(k+1:k+s1,1)=Umax;
  gamma2min(k+1:k+s1,1)=dUmin;
  gamma2max(k+1:k+s1,1)=dUmin;
end

gamma3min=zeros(s3*N2,1);
gamma3max=zeros(s3*N2,1);
for k=0:s3:(N2-1)*s3
gamma3min(k+1:k+s3,1)=Ymin;
gamma3max(k+1:k+s3,1)=Ymax;
end

C1=zeros(s1*Nu,s1);
C2=zeros(s1*Nu,s1*Nu);
for k=0:s1:(Nu-1)*s1
C1(k+1:k+s1,:)=eye(s1);
end
for k=0:s1:(Nu-1)*s1
for l=0:s1:(Nu-1)*s1
if k-l>=0
C2(k+1:k+s1,l+1:l+s1)=eye(s1);
else
C2(k+1:k+s1,l+1:l+s1)=zeros(s1);    
end
end
end
%M=[-C2;C2;eye(s1*Nu)*(-1);eye(s1*Nu);-H;H];
M=[-C2;C2];
gamma=[-gamma1min+C1*u;gamma1max-C1*u];
       %-gamma2min;gamma2max];
       %-gamma3min+F*dx+G*v_vec;gamma3max-F*dx-G*v_vec];
u_work=zeros(s1*Nu,1);
options=optimoptions('quadprog','Algorithm','interior-point-convex');
u_work=quadprog(E,f,M,gamma,[],[],dUmin,dUmax,u_work,options);
u=u_work(1:s1,1);
end
